simulink model "heater_cooler_modify"  (R2020a)
settings: Solver=VariableStepAuto  StartTime=0.0  StopTime=10.0  RelTol=1e-3
undefined symbols (not defined in the file): cooler_on, heater_on, sample5, system_off
libraries: simulink x5
settings Model: Creator=Ujwal  LastModifiedBy=Ujwal

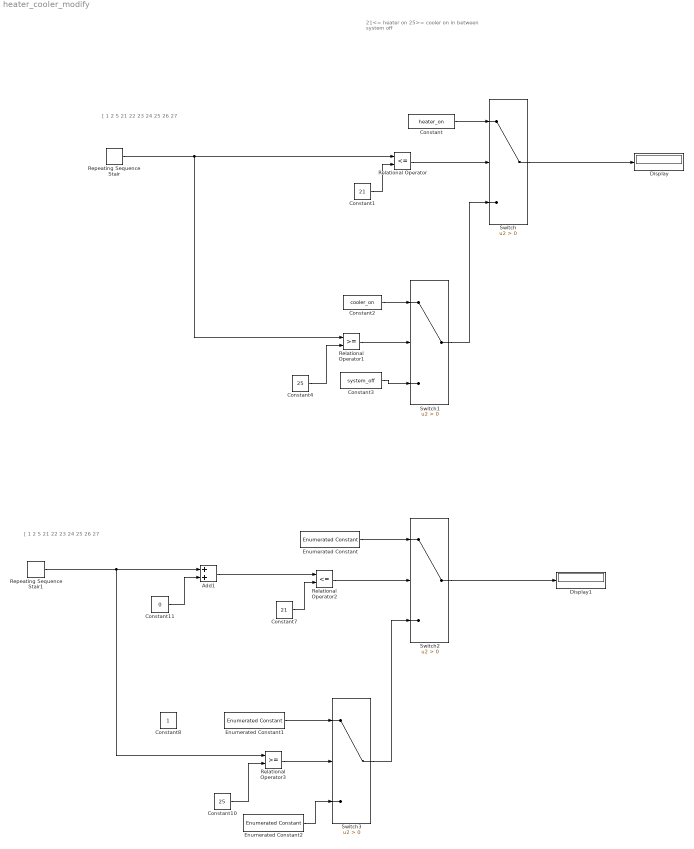
== system heater_cooler_modify ==
  note: 21<= heater on
      | 25>= cooler on
      | in between system off
  note: [ 1 2 5 21 22 23 24 25 26 27
  note: [ 1 2 5 21 22 23 24 25 26 27
  Add1 : Sum
  Constant : Constant  Value=heater_on
  Constant1 : Constant  Value=21
  Constant10 : Constant  Value=25
  Constant11 : Constant  Value=0
  Constant2 : Constant  Value=cooler_on
  Constant3 : Constant  Value=system_off
  Constant4 : Constant  Value=25
  Constant7 : Constant  Value=21
  Constant8 : Constant
  Display : Display
  Display1 : Display
  Enumerated Constant : simulink/Sources/Enumerated Constant  OutDataTypeStr=Enum: sample5  Value=sample5.heter_on  SampleTime=inf
  Enumerated Constant1 : simulink/Sources/Enumerated Constant  OutDataTypeStr=Enum: sample5  Value=sample5.cooler_on  SampleTime=inf
  Enumerated Constant2 : simulink/Sources/Enumerated Constant  OutDataTypeStr=Enum: sample5  Value=sample5.system_off  SampleTime=inf
  Relational Operator : RelationalOperator  Operator=<=  OutDataTypeStr=boolean  RndMeth=Simplest
  Relational Operator1 : RelationalOperator  OutDataTypeStr=boolean  RndMeth=Simplest
  Relational Operator2 : RelationalOperator  Operator=<=  OutDataTypeStr=boolean  RndMeth=Simplest
  Relational Operator3 : RelationalOperator  OutDataTypeStr=boolean  RndMeth=Simplest
  Repeating Sequence Stair : simulink/Sources/Repeating Sequence Stair  OutValues=[ 1 2 5 21 22 23 24 25 26 27]  tsamp=-1  OutMin=[]  OutMax=[]  OutDataTypeStr=double  OutputDataTypeScalingMode=double  OutDataType=fixdt(0,8)  ConRadixGroup=Best Precision: Vector-wise  OutScaling=2^-12
  Repeating Sequence Stair1 : simulink/Sources/Repeating Sequence Stair  OutValues=[ 1 2 5 21 22 23 24 25 26 27]  tsamp=-1  OutMin=[]  OutMax=[]  OutDataTypeStr=double  OutputDataTypeScalingMode=double  OutDataType=fixdt(0,8)  ConRadixGroup=Best Precision: Vector-wise  OutScaling=2^-12
  Switch{,1..3} (4 alike) : Switch  Criteria=u2 > Threshold
  wires:
  Relational Operator/1 -> Switch/2
  Constant/1 -> Switch/1
  Repeating Sequence Stair/1 -> Relational Operator/1, Relational Operator1/1
  Switch1/1 -> Switch/3
  Constant1/1 -> Relational Operator/2
  Relational Operator1/1 -> Switch1/2
  Constant2/1 -> Switch1/1
  Constant3/1 -> Switch1/3
  Constant4/1 -> Relational Operator1/2
  Switch/1 -> Display/1
  Relational Operator3/1 -> Switch3/2
  Constant10/1 -> Relational Operator3/2
  Repeating Sequence Stair1/1 -> Add1/1, Relational Operator3/1
  Switch2/1 -> Display1/1
  Add1/1 -> Relational Operator2/1
  Constant11/1 -> Add1/2
  Constant7/1 -> Relational Operator2/2
  Relational Operator2/1 -> Switch2/2
  Switch3/1 -> Switch2/3
  Enumerated Constant/1 -> Switch2/1
  Enumerated Constant1/1 -> Switch3/1
  Enumerated Constant2/1 -> Switch3/3
